simulink model "sistem_full_test"  (R2020b)
settings: Solver=ode45  StartTime=0.0  StopTime=10.0  MaxStep=0.01  RelTol=1e-3
undefined symbols (not defined in the file or in its folder): K_d, K_p, params, r_des
settings Model: Creator=Danil  LastModifiedBy=Danil

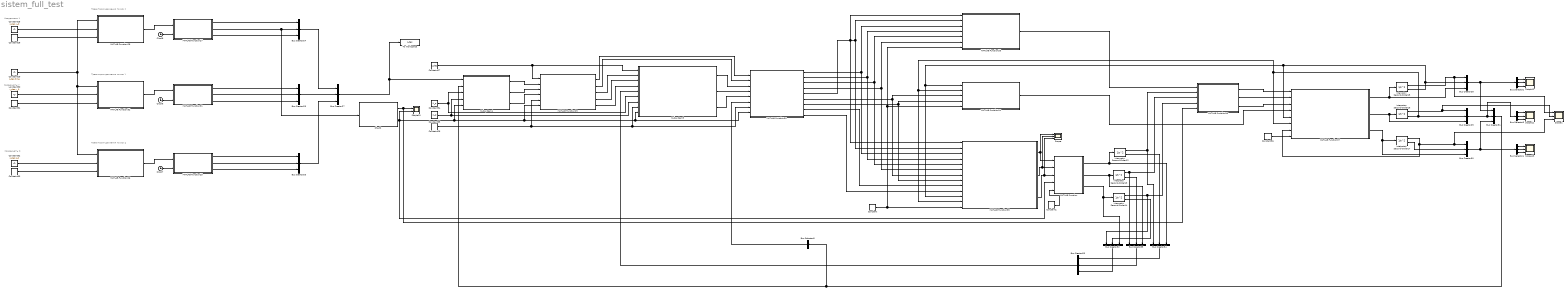
== system sistem_full_test ==
  note: Координаты X
  note: Траектория движения по оси Z
  note: Траектория движения по оси Y
  note: Траектория движения по оси X
  note: Координаты Z
  note: Координаты Y
  Bus Creator{24..35} (12 alike) : BusCreator  Inputs=3
  Bus Selector2 : BusSelector  OutputSignals=x,x_dot,x_ddot
  Bus Selector3 : BusSelector  OutputSignals=y,y_dot,y_ddot
  Bus Selector4 : BusSelector  OutputSignals=z,z_dot,z_ddot
  Bus Selector5 : BusSelector  OutputSignals=x.x_dot
  Chart2 : Stateflow chart  TreatAsAtomicUnit=on
      settings: PortSchema="{\"entries\":[{\"content\":{\"sides\":[{\"content\":{\"connectorIds\":[\"In1\"]},\"type\":\"ConnectorPlacement.EquallySpacedRectSide\",\"uuid\":\"990aaa4d-e872-427e-8bc8-a44f7de52f17\"},{\"content\":{\"connectorIds\":[\"Out2\",\"Out1\"],\"side\":\"RIGHT\"},\"type\":\"ConnectorPlacement.EquallySpacedRectSide\",\"uuid\":\"6e7ad4a8-1d47-4f26-af3c-4dfef899b5bc\"},{\"content\":{\"connectorIds\":[],\"side\":\"TOP\"},\"type\":\"ConnectorPlacement.EquallySpacedRectSide\",\"uuid\":\"20d3b10c-4783-40ca-8243-63709ccaf162\"},{\"content\":{\"connectorIds\":[],\"side\":\"HIDDEN\"},\"type\":\"ConnectorPlacement.EquallySpacedRectSide\",\"uuid\":\"c78cf433-ac9b-47b8-aa1e-24a5718d794b\"}]},\"type\":\"ConnectorPlacement.EquallySpacedConnector\",\"uuid\":\"eb598262-5703-4057-871f-faa738de211a\"}],\"packageUris\":[\"http://schema.mathworks.com/mf0/Connector/R2020b\"],\"version\":\"1.0\"}"
  Clock6 : Clock
  Clock7 : Clock
  Clock8 : Clock
  Constant{,1,26,36} (4 alike) : Constant  Value=params  OutDataTypeStr=Bus: params_bus
  Constant25 : Constant  Value=r_des.x_0
  Constant27 : Constant  Value=r_des  OutDataTypeStr=Bus: r_des_bus
  Constant28 : Constant  Value=r_des.x
  Constant29 : Constant  Value=r_des.time
  Constant30 : Constant  Value=r_des.y_0
  Constant31 : Constant  Value=r_des.y
  Constant32 : Constant  Value=r_des.z_0
  Constant33 : Constant  Value=r_des.z
  Constant34 : Constant  Value=K_p  OutDataTypeStr=Bus: K_p_bus
  Constant35 : Constant  Value=K_d  OutDataTypeStr=Bus: K_d_bus
  Integrator, Second-Order{12..17} (6 alike) : SecondOrderIntegrator
  MATLAB Function : MATLAB Function  TreatAsAtomicUnit=on
  MATLAB Function25 : MATLAB Function  TreatAsAtomicUnit=on
  MATLAB Function26 : MATLAB Function  TreatAsAtomicUnit=on
  MATLAB Function27 : MATLAB Function  TreatAsAtomicUnit=on
  MATLAB Function28 : MATLAB Function  TreatAsAtomicUnit=on
  MATLAB Function29 : MATLAB Function  TreatAsAtomicUnit=on
  MATLAB Function30 : MATLAB Function  TreatAsAtomicUnit=on
  MATLAB Function31 : MATLAB Function  TreatAsAtomicUnit=on
  MATLAB Function32 : MATLAB Function  TreatAsAtomicUnit=on
  MATLAB Function33 : MATLAB Function  TreatAsAtomicUnit=on
  MATLAB Function34 : MATLAB Function  TreatAsAtomicUnit=on
  MATLAB Function35 : MATLAB Function  TreatAsAtomicUnit=on
  MATLAB Function36 : MATLAB Function  TreatAsAtomicUnit=on
  MATLAB Function37 : MATLAB Function  TreatAsAtomicUnit=on
  Scope{,1,11..13} (5 alike) : Scope  NumInputPorts=3
  Scope10 : Scope  NumInputPorts=2
  Subsystem4 : Subsystem
  Subsystem5 : Subsystem
  To Workspace : ToWorkspace  VariableName=r_des  SaveFormat=Timeseries  SampleTime=-1
  wires:
  MATLAB Function26/1(coeff) -> MATLAB Function25/1(coeff)
  Constant31/1 -> MATLAB Function32/3(r_end)
  MATLAB Function29/5(psi_des) -> Subsystem5/4(psi_des)
  Constant27/1 -> MATLAB Function29/1(r_des), Subsystem5/1(r_des)
  MATLAB Function27/3(acc) -> Bus Creator24/3  "x_ddot"
  Bus Creator26/1 -> Bus Creator27/3  "r_z"
  Constant35/1 -> Subsystem4/4(K_d), Subsystem5/7(K_d)
  MATLAB Function27/1(pos) -> Bus Creator24/1  "x"
  MATLAB Function29/3(fi_des) -> Subsystem5/2(fi_des)
  MATLAB Function27/2(vel) -> Chart2/1(x_dot_des), Bus Creator24/2  "x_dot"
  Constant32/1 -> MATLAB Function26/2(r_0)
  Clock7/1 -> MATLAB Function25/2(clock)
  Constant34/1 -> Subsystem4/3(K_p), Subsystem5/6(K_p)
  MATLAB Function28/1(coeff) -> MATLAB Function27/1(coeff)
  Subsystem5/1(M_x) -> MATLAB Function30/3(M_x)
  Subsystem4/2(y_ddot) -> MATLAB Function29/3(y_ddot)
  Chart2/1(mode) -> Scope10/2, MATLAB Function/4(mode), MATLAB Function29/6(mode), MATLAB Function30/8(mode), Subsystem5/9(mode), Subsystem4/5(mode)
  Subsystem4/1(x_ddot) -> MATLAB Function29/2(x_ddot)
  MATLAB Function29/4(theta_des) -> Subsystem5/3(theta_des)
  Constant25/1 -> MATLAB Function28/2(r_0)
  MATLAB Function29/1(F_T) -> MATLAB Function30/1(F_T)
  Subsystem4/3(z_ddot) -> MATLAB Function29/4(z_ddot)
  MATLAB Function31/1(pos) -> Bus Creator25/1  "y"
  MATLAB Function31/3(acc) -> Bus Creator25/3  "y_ddot"
  MATLAB Function31/2(vel) -> Bus Creator25/2  "y_dot"
  Constant28/1 -> MATLAB Function28/3(r_end)
  MATLAB Function25/1(pos) -> Bus Creator26/1  "z"
  Bus Creator24/1 -> Bus Creator27/1  "r_x"
  MATLAB Function32/1(coeff) -> MATLAB Function31/1(coeff)
  MATLAB Function25/2(vel) -> Bus Creator26/2  "z_dot"
  Subsystem5/3(M_z) -> MATLAB Function30/5(M_z)
  Constant30/1 -> MATLAB Function32/2(r_0)
  Constant33/1 -> MATLAB Function26/3(r_end)
  MATLAB Function25/3(acc) -> Bus Creator26/3  "z_ddot"
  Bus Creator25/1 -> Bus Creator27/2  "r_y"
  Clock8/1 -> MATLAB Function27/2(clock)
  Bus Creator27/1 -> To Workspace/1, Subsystem4/1(r_des)
  Constant26/1 -> MATLAB Function29/5(params), Subsystem5/8(params), MATLAB Function30/7(params)
  Subsystem5/2(M_y) -> MATLAB Function30/4(M_y)
  Clock6/1 -> MATLAB Function31/2(clock)
  Constant29/1 -> MATLAB Function26/1(t), MATLAB Function32/1(t), MATLAB Function28/1(t)
  MATLAB Function29/2(Y) -> MATLAB Function30/2(Y)
  MATLAB Function/1(fi_ddot) -> "Integrator, Second-Order12"/1, Bus Creator34/3  "fi_ddot"
  MATLAB Function37/1(x_ddot) -> Bus Creator28/3, "Integrator, Second-Order15"/1
  MATLAB Function37/3(z_ddot) -> Bus Creator30/3, "Integrator, Second-Order17"/1
  MATLAB Function30/5(w) -> MATLAB Function35/2(w_R), MATLAB Function33/2(w_R), MATLAB Function33/1(w_L), MATLAB Function35/1(w_L)
  MATLAB Function/3(psi_ddot) -> Bus Creator32/3, "Integrator, Second-Order14"/1  "psi_ddot"
  MATLAB Function36/1(F_x) -> MATLAB Function37/1(F_x)
  MATLAB Function37/2(y_ddot) -> Bus Creator29/3, "Integrator, Second-Order16"/1
  MATLAB Function36/3(F_z) -> MATLAB Function37/3(F_z)
  "Integrator, Second-Order16"/2 -> MATLAB Function37/6(y_dot), MATLAB Function34/2(y_dot), MATLAB Function35/12(y_dot), Bus Creator29/2  "y_dot"
  MATLAB Function30/1(alpha_1) -> MATLAB Function35/3(alpha_1), MATLAB Function33/3(alpha_1)
  MATLAB Function30/6(alpha_L) -> MATLAB Function35/7(alpha_L), MATLAB Function34/3(alpha_L)
  MATLAB Function30/4(alpha_4) -> MATLAB Function35/6(alpha_4), MATLAB Function33/6(alpha_4)
  MATLAB Function/2(theta_ddot) -> Bus Creator35/3, "Integrator, Second-Order13"/1  "theta_ddot"
  "Integrator, Second-Order15"/2 -> Bus Creator28/2, MATLAB Function37/5(x_dot), MATLAB Function34/1(x_dot), MATLAB Function35/11(x_dot)  "x_dot"
  MATLAB Function34/1(Y) -> MATLAB Function37/4(Y)
  Constant/1 -> MATLAB Function35/13(params), MATLAB Function34/5(params), MATLAB Function33/7(params)
  Constant36/1 -> MATLAB Function37/8(params)
  "Integrator, Second-Order12"/1 -> MATLAB Function36/2(fi), Bus Creator34/1  "fi"
  MATLAB Function33/1(F) -> MATLAB Function36/1(F)
  MATLAB Function30/2(alpha_2) -> MATLAB Function35/4(alpha_2), MATLAB Function33/4(alpha_2)
  MATLAB Function30/9(alpha_F) -> MATLAB Function35/10(alpha_F)
  MATLAB Function30/8(alpha_H) -> MATLAB Function35/9(alpha_H)
  MATLAB Function36/2(F_y) -> MATLAB Function37/2(F_y)
  MATLAB Function30/7(alpha_R) -> MATLAB Function35/8(alpha_R), MATLAB Function34/4(alpha_R)
  MATLAB Function30/3(alpha_3) -> MATLAB Function35/5(alpha_3), MATLAB Function33/5(alpha_3)
  Chart2/2(sigma) -> MATLAB Function36/5(sigma), Scope10/1
  "Integrator, Second-Order14"/1 -> Bus Creator32/1, MATLAB Function36/4(psi)  "psi"
  "Integrator, Second-Order17"/1 -> Scope1/3, Bus Creator30/1, MATLAB Function37/7(z_dot)  "z"
  "Integrator, Second-Order13"/1 -> MATLAB Function36/3(theta), Bus Creator35/1  "theta"
  Bus Creator28/1 -> Bus Creator31/1, Bus Selector2/1  "x"
  Bus Creator29/1 -> Bus Selector3/1, Bus Creator31/2  "y"
  Bus Creator30/1 -> Bus Selector4/1, Bus Creator31/3  "z"
  Bus Creator32/1 -> Bus Creator33/3  "psi"
  Bus Creator34/1 -> Bus Creator33/1  "fi"
  Bus Creator35/1 -> Bus Creator33/2  "theta"
  "Integrator, Second-Order15"/1 -> Scope1/1, Bus Creator28/1  "x"
  "Integrator, Second-Order16"/1 -> Bus Creator29/1, Scope1/2  "y"
  "Integrator, Second-Order17"/2 -> Bus Creator30/2  "z_dot"
  Bus Selector3/2 -> Scope11/2  "<y_dot>"
  Bus Selector3/3 -> Scope11/3  "<y_ddot>"
  Bus Selector3/1 -> Scope11/1  "<y>"
  Bus Selector4/2 -> Scope13/2  "<z_dot>"
  Bus Selector4/3 -> Scope13/3  "<z_ddot>"
  Bus Selector4/1 -> Scope13/1  "<z>"
  Bus Selector2/2 -> Scope12/2  "<x_dot>"
  Bus Selector2/3 -> Scope12/3  "<x_ddot>"
  Bus Selector2/1 -> Scope12/1  "<x>"
  "Integrator, Second-Order12"/2 -> Bus Creator34/2  "fi_dot"
  "Integrator, Second-Order13"/2 -> Bus Creator35/2  "theta_dot"
  "Integrator, Second-Order14"/2 -> Bus Creator32/2  "psi_dot"
  Bus Creator31/1 -> Bus Selector5/1, Subsystem4/2(r)
  Bus Creator33/1 -> Subsystem5/5(r)
  Bus Selector5/1 -> MATLAB Function30/6(x_dot)  "<x_dot>"
  MATLAB Function35/1(M_x) -> MATLAB Function/1(M_x), Scope/1
  MATLAB Function35/2(M_y) -> Scope/2, MATLAB Function/2(M_y)
  MATLAB Function35/3(M_z) -> Scope/3, MATLAB Function/3(M_z)
  Constant1/1 -> MATLAB Function/5(params)

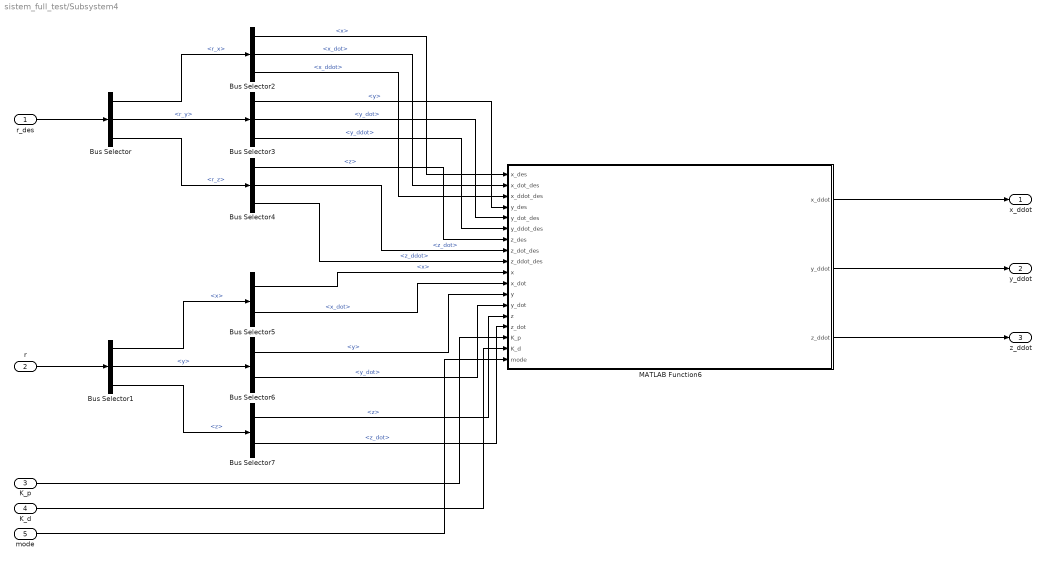
== system sistem_full_test/Subsystem4 ==
  r_des : Inport
  r : Inport  Port=2
  K_p : Inport  Port=3
  K_d : Inport  Port=4
  mode : Inport  Port=5
  Bus Selector : BusSelector  OutputSignals=r_x,r_y,r_z
  Bus Selector1 : BusSelector  OutputSignals=x,y,z
  Bus Selector2 : BusSelector  OutputSignals=x,x_dot,x_ddot
  Bus Selector3 : BusSelector  OutputSignals=y,y_dot,y_ddot
  Bus Selector4 : BusSelector  OutputSignals=z,z_dot,z_ddot
  Bus Selector5 : BusSelector  OutputSignals=x,x_dot
  Bus Selector6 : BusSelector  OutputSignals=y,y_dot
  Bus Selector7 : BusSelector  OutputSignals=z,z_dot
  MATLAB Function6 : MATLAB Function  TreatAsAtomicUnit=on
  x_ddot : Outport
  y_ddot : Outport  Port=2
  z_ddot : Outport  Port=3
  wires:
  Bus Selector3/1 -> MATLAB Function6/4(y_des)  "<y>"
  Bus Selector4/3 -> MATLAB Function6/9(z_ddot_des)  "<z_ddot>"
  Bus Selector4/1 -> MATLAB Function6/7(z_des)  "<z>"
  Bus Selector/1 -> Bus Selector2/1  "<r_x>"
  Bus Selector5/2 -> MATLAB Function6/11(x_dot)  "<x_dot>"
  Bus Selector3/2 -> MATLAB Function6/5(y_dot_des)  "<y_dot>"
  Bus Selector/3 -> Bus Selector4/1  "<r_z>"
  r/1 -> Bus Selector1/1
  r_des/1 -> Bus Selector/1
  Bus Selector2/1 -> MATLAB Function6/1(x_des)  "<x>"
  Bus Selector5/1 -> MATLAB Function6/10(x)  "<x>"
  MATLAB Function6/2(y_ddot) -> y_ddot/1
  MATLAB Function6/3(z_ddot) -> z_ddot/1
  K_d/1 -> MATLAB Function6/17(K_d)
  K_p/1 -> MATLAB Function6/16(K_p)
  Bus Selector1/3 -> Bus Selector7/1  "<z>"
  Bus Selector2/2 -> MATLAB Function6/2(x_dot_des)  "<x_dot>"
  Bus Selector7/2 -> MATLAB Function6/15(z_dot)  "<z_dot>"
  MATLAB Function6/1(x_ddot) -> x_ddot/1
  Bus Selector6/1 -> MATLAB Function6/12(y)  "<y>"
  Bus Selector7/1 -> MATLAB Function6/14(z)  "<z>"
  Bus Selector4/2 -> MATLAB Function6/8(z_dot_des)  "<z_dot>"
  Bus Selector2/3 -> MATLAB Function6/3(x_ddot_des)  "<x_ddot>"
  Bus Selector1/1 -> Bus Selector5/1  "<x>"
  Bus Selector1/2 -> Bus Selector6/1  "<y>"
  Bus Selector6/2 -> MATLAB Function6/13(y_dot)  "<y_dot>"
  Bus Selector3/3 -> MATLAB Function6/6(y_ddot_des)  "<y_ddot>"
  Bus Selector/2 -> Bus Selector3/1  "<r_y>"
  mode/1 -> MATLAB Function6/18(mode)

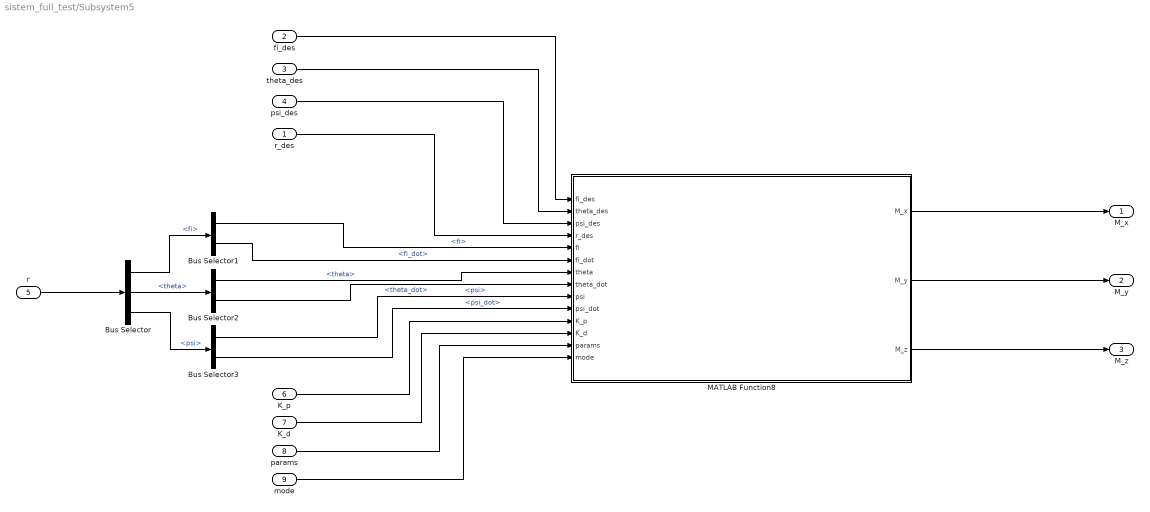
== system sistem_full_test/Subsystem5 ==
  r_des : Inport
  fi_des : Inport  Port=2
  theta_des : Inport  Port=3
  psi_des : Inport  Port=4
  r : Inport  Port=5
  K_p : Inport  Port=6
  K_d : Inport  Port=7
  params : Inport  Port=8
  mode : Inport  Port=9
  Bus Selector : BusSelector  OutputSignals=fi,theta,psi
  Bus Selector1 : BusSelector  OutputSignals=fi,fi_dot
  Bus Selector2 : BusSelector  OutputSignals=theta,theta_dot
  Bus Selector3 : BusSelector  OutputSignals=psi,psi_dot
  MATLAB Function8 : MATLAB Function  TreatAsAtomicUnit=on
  M_x : Outport
  M_y : Outport  Port=2
  M_z : Outport  Port=3
  wires:
  Bus Selector3/1 -> MATLAB Function8/9(psi)  "<psi>"
  Bus Selector1/2 -> MATLAB Function8/6(fi_dot)  "<fi_dot>"
  Bus Selector/1 -> Bus Selector1/1  "<fi>"
  Bus Selector1/1 -> MATLAB Function8/5(fi)  "<fi>"
  r/1 -> Bus Selector/1
  MATLAB Function8/3(M_z) -> M_z/1
  MATLAB Function8/1(M_x) -> M_x/1
  MATLAB Function8/2(M_y) -> M_y/1
  Bus Selector2/2 -> MATLAB Function8/8(theta_dot)  "<theta_dot>"
  K_p/1 -> MATLAB Function8/11(K_p)
  Bus Selector2/1 -> MATLAB Function8/7(theta)  "<theta>"
  Bus Selector/2 -> Bus Selector2/1  "<theta>"
  r_des/1 -> MATLAB Function8/4(r_des)
  params/1 -> MATLAB Function8/13(params)
  psi_des/1 -> MATLAB Function8/3(psi_des)
  fi_des/1 -> MATLAB Function8/1(fi_des)
  K_d/1 -> MATLAB Function8/12(K_d)
  theta_des/1 -> MATLAB Function8/2(theta_des)
  Bus Selector3/2 -> MATLAB Function8/10(psi_dot)  "<psi_dot>"
  Bus Selector/3 -> Bus Selector3/1  "<psi>"
  mode/1 -> MATLAB Function8/14(mode)

== matlab function sistem_full_test/MATLAB Function30 ==
  data: alpha_1 output; alpha_2 output; alpha_3 output; alpha_4 output; F_T input; Y input; w output; M_x input; M_y input; M_z input; x_dot input; params input; alpha_L output; alpha_R output; alpha_H output; alpha_F output; mode input
function [alpha_1, alpha_2, alpha_3, alpha_4, w, alpha_L, alpha_R, alpha_H, alpha_F] = fcn(F_T, Y, M_x, M_y, M_z, x_dot, params, mode)

if mode == 0
    
    alpha_1 = (1 / (4 * params.k_Y)) * (F_T + M_x + M_y + M_z) - 7;
    alpha_2 = (1 / (4 * params.k_Y)) * (F_T + M_x - M_y - M_z);
    alpha_3 = (1 / (4 * params.k_Y)) * (F_T - M_x + M_y - M_z) - 7;
    alpha_4 = (1 / (4 * params.k_Y)) * (F_T - M_x - M_y + M_z);
    
    w = params.w_0;
    alpha_L = -7;
    alpha_R = -7;
    alpha_H = 0;
    alpha_F = 0;
    
elseif mode == 1
    
    alpha_1 = 7.5;
    alpha_2 = 7.5;
    alpha_3 = 7.5;
    alpha_4 = 7.5;

    w = (50000 * F_T + 245100) / 77;

    alpha_L = (500 * M_x + 500 * Y + 102201 * params.S_k * params.rho - 14630 * params.S_k * params.rho * x_dot) / (30 * params.S_k * params.rho * (70 * x_dot - 489));
    alpha_R = - (500 * M_x - 500 * Y - 102201 * params.S_k * params.rho + 14630 * params.S_k * params.rho * x_dot) / (30 * params.S_k * params.rho * (70 * x_dot - 489));
    alpha_H = (125 * M_y) / (3 * params.S_h * params.rho * (70 * x_dot - 489));
    alpha_F = (125 * M_z) / (3 * params.S_f * params.rho * (70 * x_dot - 489));
    
else
    
    alpha_1 = (1 / (4 * params.k_Y)) * (F_T + M_x + M_y + M_z) - 7;
    alpha_2 = (1 / (4 * params.k_Y)) * (F_T + M_x - M_y - M_z);
    alpha_3 = (1 / (4 * params.k_Y)) * (F_T - M_x + M_y - M_z) - 7;
    alpha_4 = (1 / (4 * params.k_Y)) * (F_T - M_x - M_y + M_z);
    
    w = params.w_0;
    alpha_L = -7;
    alpha_R = -7;
    alpha_H = 0;
    alpha_F = 0;
    
end

== matlab function sistem_full_test/MATLAB Function31 ==
  data: coeff input; pos output; clock input; vel output; acc output
function [pos, vel, acc] = trajectories_calculation(coeff, clock)

T_p = [clock^5      clock^4     clock^3     clock^2     clock   1]';
T_v = [5*clock^4    4*clock^3   3*clock^2   2*clock     1       0]';
T_a = [20*clock^3   12*clock^2  6*clock     2           0       0]';

pos = sum(coeff.*T_p);
vel = sum(coeff.*T_v);
acc = sum(coeff.*T_a);

== matlab function sistem_full_test/MATLAB Function32 ==
  data: t input; coeff output; r_0 input; r_end input
function coeff  = calculation_coefficients(t, r_0, r_end)

x_0 = r_0;
x_dot_0 = 0;
x_ddot_0 = 0;

x_des = r_end;
x_dot_des = 0;
x_ddot_des = 0;

waypoints = [x_0    x_dot_0     x_ddot_0;
             x_des  x_dot_des   x_ddot_des]';
t = [0 t];

time_size = size(t);
n = 0;
%T = linspace(0, time_size(2) - 1, point(2));


border_conditions_sigm = reshape(waypoints(:, n + 1 : n + 2),1,[]);
%disp(border_conditions_sigm)

coeff = zeros(6, 1);

parameters = [1 * (t(n + 1) ^ 5), 1 * (t(n + 1) ^ 4), 1 * (t(n + 1) ^ 3), 1 * (t(n + 1) ^ 2), 1 * (t(n + 1) ^ 1), 1 * (t(n + 1) ^ 0);
              5 * (t(n + 1) ^ 4), 4 * (t(n + 1) ^ 3), 3 * (t(n + 1) ^ 2), 2 * (t(n + 1) ^ 1), 1 * (t(n + 1) ^ 0), 0 * (t(n + 1) ^ 0);
              20 * (t(n + 1) ^ 3), 12 * (t(n + 1) ^ 2), 6 * (t(n + 1) ^ 1), 2 * (t(n + 1) ^ 0), 0 * (t(n + 1) ^ 0), 0 * (t(n + 1) ^ 0);
              1 * (t(n + 2) ^ 5), 1 * (t(n + 2) ^ 4), 1 * (t(n + 2) ^ 3), 1 * (t(n + 2) ^ 2), 1 * (t(n + 2) ^ 1), 1 * (t(n + 2) ^ 0);
              5 * (t(n + 2) ^ 4), 4 * (t(n + 2) ^ 3), 3 * (t(n + 2) ^ 2), 2 * (t(n + 2) ^ 1), 1 * (t(n + 2) ^ 0), 0 * (t(n + 2) ^ 0);
              20 * (t(n + 2) ^ 3), 12 * (t(n + 2) ^ 2), 6 * (t(n + 2) ^ 1), 2 * (t(n + 2) ^ 0), 0 * (t(n + 2) ^ 0), 0 * (t(n + 2) ^ 0)];

coeff = inv(parameters) * border_conditions_sigm';

== matlab function sistem_full_test/Subsystem4/MATLAB Function6 ==
  data: x_des input; x_ddot output; x_dot_des input; x_ddot_des input; y_des input; y_dot_des input; y_ddot_des input; z_des input; z_dot_des input; z_ddot_des input; x input; x_dot input; y input; y_dot input; z input; z_dot input; K_p input; K_d input; y_ddot output; z_ddot output; mode input
function [x_ddot,y_ddot,z_ddot] = fcn(x_des, x_dot_des, x_ddot_des, y_des, y_dot_des, y_ddot_des, z_des, z_dot_des, z_ddot_des, ...
                                      x, x_dot, y, y_dot, z, z_dot, K_p, K_d, mode)

if mode == 0
    
    x_ddot = x_ddot_des + abs(K_d.ver.x) * (x_dot_des - x_dot) + abs(K_p.ver.x) * (x_des - x);
    y_ddot = y_ddot_des + abs(K_d.ver.y) * (y_dot_des - y_dot) + abs(K_p.ver.y) * (y_des - y);
    z_ddot = z_ddot_des + abs(K_d.ver.z) * (z_dot_des - z_dot) + abs(K_p.ver.z) * (z_des - z);

elseif mode == 1
    
    x_ddot = x_ddot_des + abs(K_d.hor.x) * (x_dot_des - x_dot) + abs(K_p.hor.x) * (x_des - x);
    y_ddot = y_ddot_des + abs(K_d.hor.y) * (y_dot_des - y_dot) + abs(K_p.hor.y) * (y_des - y);
    z_ddot = z_ddot_des + abs(K_d.hor.z) * (z_dot_des - z_dot) + abs(K_p.hor.z) * (z_des - z);
    
else
    
    x_ddot = x_ddot_des + abs(K_d.ver.x) * (x_dot_des - x_dot) + abs(K_p.ver.x) * (x_des - x);
    y_ddot = y_ddot_des + abs(K_d.ver.y) * (y_dot_des - y_dot) + abs(K_p.ver.y) * (y_des - y);
    z_ddot = z_ddot_des + abs(K_d.ver.z) * (z_dot_des - z_dot) + abs(K_p.ver.z) * (z_des - z);
    
end

== matlab function sistem_full_test/Subsystem5/MATLAB Function8 ==
  data: fi_des input; theta_des input; psi_des input; r_des input; fi input; fi_dot input; theta input; theta_dot input; psi input; psi_dot input; M_x output; K_p input; K_d input; params input; M_y output; M_z output; mode input
function [M_x, M_y, M_z] = fcn(fi_des, theta_des, psi_des, r_des, fi, fi_dot, theta, theta_dot, psi, psi_dot, K_p, K_d, params, mode)

if mode == 0

    M_x = (params.ver.J_xx / params.ver.L_x) * (r_des.fi_ddot + abs(K_d.ver.fi) * (r_des.fi_dot - fi_dot) + abs(K_p.ver.fi) * (fi_des - fi));
    M_y = (params.ver.J_yy / params.ver.L_y) * (r_des.theta_ddot + abs(K_d.ver.theta) * (r_des.theta_dot - theta_dot) + abs(K_p.ver.theta) * (theta_des - theta));
    M_z = (params.ver.J_zz / params.ver.L_z) * (r_des.psi_ddot + abs(K_d.ver.psi) * (r_des.psi_dot - psi_dot) + abs(K_p.ver.psi) * (psi_des - psi));
    
elseif mode == 1
    
    M_x = (params.hor.J_xx / params.hor.L_x) * (r_des.fi_ddot + abs(K_d.hor.fi) * (r_des.fi_dot - fi_dot) + abs(K_p.hor.fi) * (fi_des - fi));
    M_y = (params.hor.J_yy / params.hor.L_y) * (r_des.theta_ddot + abs(K_d.hor.theta) * (r_des.theta_dot - theta_dot) + abs(K_p.hor.theta) * (theta_des - theta));
    M_z = (params.hor.J_zz / params.hor.L_z) * (r_des.psi_ddot + abs(K_d.hor.psi) * (r_des.psi_dot - psi_dot) + abs(K_p.hor.psi) * (psi_des - psi));
    
else 
    
    M_x = (params.ver.J_xx / params.ver.L_x) * (r_des.fi_ddot + abs(K_d.ver.fi) * (r_des.fi_dot - fi_dot) + abs(K_p.ver.fi) * (fi_des - fi));
    M_y = (params.ver.J_yy / params.ver.L_y) * (r_des.theta_ddot + abs(K_d.ver.theta) * (r_des.theta_dot - theta_dot) + abs(K_p.ver.theta) * (theta_des - theta));
    M_z = (params.ver.J_zz / params.ver.L_z) * (r_des.psi_ddot + abs(K_d.ver.psi) * (r_des.psi_dot - psi_dot) + abs(K_p.ver.psi) * (psi_des - psi));
    
end

== matlab function sistem_full_test/MATLAB Function33 ==
  data: w_L input; F output; w_R input; alpha_1 input; alpha_2 input; alpha_3 input; alpha_4 input; params input
function F  = fcn(w_L, w_R, alpha_1, alpha_2, alpha_3, alpha_4, params)

alpha_L = alpha_1 + alpha_2;
alpha_R = alpha_3 + alpha_4;

C_Y_L = params.a_l * alpha_L^2 + params.b_l * alpha_L + params.c_l;
C_Y_R = params.a_l * alpha_R^2 + params.b_l * alpha_R + params.c_l;

F = (3/2) * params.rho * params.S_l * (C_Y_L * w_L^2 + C_Y_R * w_R^2);

== matlab function sistem_full_test/MATLAB Function34 ==
  data: x_dot input; y_dot input; alpha_L input; alpha_R input; params input; Y output
function Y = fcn(x_dot, y_dot, alpha_L, alpha_R, params)

C_y_L = params.a_k * alpha_L^2 + params.b_k * alpha_L + params.c_k;
C_y_R = params.a_k * alpha_R^2 + params.b_k * alpha_R + params.c_k;

Y = (1 / 2) * params.rho * (x_dot^2 + y_dot^2) * params.S_k * (C_y_L + C_y_R);

== matlab function sistem_full_test/MATLAB Function35 ==
  data: w_L input; w_R input; alpha_1 input; alpha_2 input; alpha_3 input; alpha_4 input; alpha_L input; alpha_R input; alpha_H input; alpha_F input; x_dot input; y_dot input; M_x output; M_y output; M_z output; params input
function [M_x, M_y, M_z] = fcn(w_L, w_R, alpha_1, alpha_2, alpha_3, alpha_4, ...
                               alpha_L, alpha_R, alpha_H, alpha_F, x_dot, y_dot, params)

C_y_L_l_x = params.a_l * (alpha_1 + alpha_2)^2 + params.b_l * (alpha_1 + alpha_2) + params.c_l;
C_y_R_l_x = params.a_l * (alpha_3 + alpha_4)^2 + params.b_l * (alpha_3 + alpha_4) + params.c_l;

C_y_L_l_yz = params.a_l * (alpha_1 - alpha_2)^2 + params.b_l * (alpha_1 - alpha_2) + params.c_l;
C_y_R_l_yz = params.a_l * (alpha_3 - alpha_4)^2 + params.b_l * (alpha_3 - alpha_4) + params.c_l;

C_y_L_k = params.a_k * alpha_L^2 + params.b_k * alpha_L + params.c_k;
C_y_R_k = params.a_k * alpha_R^2 + params.b_k * alpha_R + params.c_k;

C_y_H = params.a_h * alpha_H^3 + params.b_h * alpha_H^2 + params.c_h * alpha_H + params.d_h;
C_y_F = params.a_f * alpha_F^3 + params.b_f * alpha_F^2 + params.c_f * alpha_F + params.d_f;

M_x = ((3 / 2) * params.rho * params.S_l * (C_y_L_l_x * w_L^2 - C_y_R_l_x * w_R^2)) + ...
      ((1 / 2) * params.rho * params.S_k * (x_dot^2 + y_dot^2) * (C_y_L_k - C_y_R_k));
  
M_y = ((3 / 2) * params.rho * params.S_l * (C_y_L_l_yz * w_L^2 + C_y_R_l_yz * w_R^2)) + ...
      ((1 / 2) * C_y_H * params.rho * params.S_h * (x_dot^2 + y_dot^2));
  
M_z = ((3 / 2) * params.rho * params.S_l * (C_y_L_l_yz * w_L^2 - C_y_R_l_yz * w_R^2)) + ...
      ((1 / 2) * C_y_F * params.rho * params.S_f * (x_dot^2 + y_dot^2));

== matlab function sistem_full_test/MATLAB Function36 ==
  data: F input; F_x output; fi input; theta input; psi input; F_y output; F_z output; sigma input
function [F_x, F_y, F_z] = fcn(F, fi, theta, psi, sigma)

sigma = sigma * pi / 180;

F_x = F * sin(sigma) * (cos(psi) * sin(theta) + cos(theta) * sin(fi) * sin(psi)) + F * cos(sigma) * (cos(psi) * cos(theta));
F_y = F * sin(sigma) * (sin(psi) * sin(theta) - cos(psi) * cos(theta) * sin(fi)) + F * cos(sigma) * (cos(fi) * sin(psi) + cos(psi) * sin(fi) * sin(theta));
F_z = F * sin(sigma) * (cos(fi) * cos(theta)) + F * cos(sigma) * (sin(fi) * sin(psi) - cos(fi) * cos(psi) * sin(theta));

== matlab function sistem_full_test/MATLAB Function37 ==
  data: F_x input; x_ddot output; F_y input; F_z input; Y input; x_dot input; y_dot input; z_dot input; params input; y_ddot output; z_ddot output
function [x_ddot, y_ddot, z_ddot] = fcn(F_x, F_y, F_z, Y, x_dot, y_dot, z_dot, params)

x_ddot = (1 / params.m) * (F_x - params.k_x * x_dot);
y_ddot = (1 / params.m) * (F_y - params.k_y * y_dot);
z_ddot = (1 / params.m) * (F_z + Y - params.k_z * z_dot - params.m * params.g);

== matlab function sistem_full_test/MATLAB Function ==
  data: M_x input; fi_ddot output; M_y input; M_z input; mode input; params input; theta_ddot output; psi_ddot output
function [fi_ddot, theta_ddot, psi_ddot] = fcn(M_x, M_y, M_z, mode, params)

if mode == 0
    
    fi_ddot = (params.ver.L_x / params.ver.J_xx) * M_x;
    theta_ddot = (params.ver.L_y / params.ver.J_yy) * M_y;
    psi_ddot = (params.ver.L_z / params.ver.J_zz) * M_z;
    
elseif mode == 1
    
    fi_ddot = (params.hor.L_x / params.hor.J_xx) * M_x;
    theta_ddot = (params.hor.L_y / params.hor.J_yy) * M_y;
    psi_ddot = (params.hor.L_z / params.hor.J_zz) * M_z;
    
else
    
    fi_ddot = (params.ver.L_x / params.ver.J_xx) * M_x;
    theta_ddot = (params.ver.L_y / params.ver.J_yy) * M_y;
    psi_ddot = (params.ver.L_z / params.ver.J_zz) * M_z;
    
end

== stateflow chart sistem_full_test/Chart2 ==
  state Vertical_flight
    mode = 0
    sigma = 90
  state Horizontal_flight
    mode = 1
    sigma = 0
  (default) -> Vertical_flight
  Horizontal_flight -> Vertical_flight : [x_dot_des < 14.1]
  Vertical_flight -> Horizontal_flight : [x_dot_des > 14.1]
  data: mode output; x_dot_des input; sigma output

== matlab function sistem_full_test/MATLAB Function25 ==
  data: coeff input; pos output; clock input; vel output; acc output
function [pos, vel, acc] = trajectories_calculation(coeff, clock)

T_p = [clock^5      clock^4     clock^3     clock^2     clock   1]';
T_v = [5*clock^4    4*clock^3   3*clock^2   2*clock     1       0]';
T_a = [20*clock^3   12*clock^2  6*clock     2           0       0]';

pos = sum(coeff.*T_p);
vel = sum(coeff.*T_v);
acc = sum(coeff.*T_a);

== matlab function sistem_full_test/MATLAB Function26 ==
  data: t input; coeff output; r_0 input; r_end input
function coeff  = calculation_coefficients(t, r_0, r_end)

x_0 = r_0;
x_dot_0 = 0;
x_ddot_0 = 0;

x_des = r_end;
x_dot_des = 0;
x_ddot_des = 0;

waypoints = [x_0    x_dot_0     x_ddot_0;
             x_des  x_dot_des   x_ddot_des]';
t = [0 t];

time_size = size(t);
n = 0;
%T = linspace(0, time_size(2) - 1, point(2));


border_conditions_sigm = reshape(waypoints(:, n + 1 : n + 2),1,[]);
%disp(border_conditions_sigm)

coeff = zeros(6, 1);

parameters = [1 * (t(n + 1) ^ 5), 1 * (t(n + 1) ^ 4), 1 * (t(n + 1) ^ 3), 1 * (t(n + 1) ^ 2), 1 * (t(n + 1) ^ 1), 1 * (t(n + 1) ^ 0);
              5 * (t(n + 1) ^ 4), 4 * (t(n + 1) ^ 3), 3 * (t(n + 1) ^ 2), 2 * (t(n + 1) ^ 1), 1 * (t(n + 1) ^ 0), 0 * (t(n + 1) ^ 0);
              20 * (t(n + 1) ^ 3), 12 * (t(n + 1) ^ 2), 6 * (t(n + 1) ^ 1), 2 * (t(n + 1) ^ 0), 0 * (t(n + 1) ^ 0), 0 * (t(n + 1) ^ 0);
              1 * (t(n + 2) ^ 5), 1 * (t(n + 2) ^ 4), 1 * (t(n + 2) ^ 3), 1 * (t(n + 2) ^ 2), 1 * (t(n + 2) ^ 1), 1 * (t(n + 2) ^ 0);
              5 * (t(n + 2) ^ 4), 4 * (t(n + 2) ^ 3), 3 * (t(n + 2) ^ 2), 2 * (t(n + 2) ^ 1), 1 * (t(n + 2) ^ 0), 0 * (t(n + 2) ^ 0);
              20 * (t(n + 2) ^ 3), 12 * (t(n + 2) ^ 2), 6 * (t(n + 2) ^ 1), 2 * (t(n + 2) ^ 0), 0 * (t(n + 2) ^ 0), 0 * (t(n + 2) ^ 0)];

coeff = inv(parameters) * border_conditions_sigm';

== matlab function sistem_full_test/MATLAB Function27 ==
  data: coeff input; pos output; clock input; vel output; acc output
function [pos, vel, acc] = trajectories_calculation(coeff, clock)

T_p = [clock^5      clock^4     clock^3     clock^2     clock   1]';
T_v = [5*clock^4    4*clock^3   3*clock^2   2*clock     1       0]';
T_a = [20*clock^3   12*clock^2  6*clock     2           0       0]';

pos = sum(coeff.*T_p);
vel = sum(coeff.*T_v);
acc = sum(coeff.*T_a);

== matlab function sistem_full_test/MATLAB Function28 ==
  data: t input; coeff output; r_0 input; r_end input
function coeff  = calculation_coefficients(t, r_0, r_end)

x_0 = r_0;
x_dot_0 = 0;
x_ddot_0 = 0;

x_des = r_end;
x_dot_des = 0;
x_ddot_des = 0;

waypoints = [x_0    x_dot_0     x_ddot_0;
             x_des  x_dot_des   x_ddot_des]';
t = [0 t];

time_size = size(t);
n = 0;
%T = linspace(0, time_size(2) - 1, point(2));


border_conditions_sigm = reshape(waypoints(:, n + 1 : n + 2),1,[]);
%disp(border_conditions_sigm)

coeff = zeros(6, 1);

parameters = [1 * (t(n + 1) ^ 5), 1 * (t(n + 1) ^ 4), 1 * (t(n + 1) ^ 3), 1 * (t(n + 1) ^ 2), 1 * (t(n + 1) ^ 1), 1 * (t(n + 1) ^ 0);
              5 * (t(n + 1) ^ 4), 4 * (t(n + 1) ^ 3), 3 * (t(n + 1) ^ 2), 2 * (t(n + 1) ^ 1), 1 * (t(n + 1) ^ 0), 0 * (t(n + 1) ^ 0);
              20 * (t(n + 1) ^ 3), 12 * (t(n + 1) ^ 2), 6 * (t(n + 1) ^ 1), 2 * (t(n + 1) ^ 0), 0 * (t(n + 1) ^ 0), 0 * (t(n + 1) ^ 0);
              1 * (t(n + 2) ^ 5), 1 * (t(n + 2) ^ 4), 1 * (t(n + 2) ^ 3), 1 * (t(n + 2) ^ 2), 1 * (t(n + 2) ^ 1), 1 * (t(n + 2) ^ 0);
              5 * (t(n + 2) ^ 4), 4 * (t(n + 2) ^ 3), 3 * (t(n + 2) ^ 2), 2 * (t(n + 2) ^ 1), 1 * (t(n + 2) ^ 0), 0 * (t(n + 2) ^ 0);
              20 * (t(n + 2) ^ 3), 12 * (t(n + 2) ^ 2), 6 * (t(n + 2) ^ 1), 2 * (t(n + 2) ^ 0), 0 * (t(n + 2) ^ 0), 0 * (t(n + 2) ^ 0)];

coeff = inv(parameters) * border_conditions_sigm';

== matlab function sistem_full_test/MATLAB Function29 ==
  data: r_des input; F_T output; Y output; fi_des output; x_ddot input; y_ddot input; z_ddot input; params input; mode input; theta_des output; psi_des output
function [F_T, Y, fi_des, theta_des, psi_des] = fcn(r_des, x_ddot, y_ddot, z_ddot, params, mode)

if mode == 0
    
    F_T = params.m * (z_ddot + params.g);
    Y = 0;

    fi_des = (1 / params.g) * (x_ddot * sin(r_des.psi) - y_ddot * cos(r_des.psi));
    theta_des = (1 / params.g) * (x_ddot * cos(r_des.psi) + y_ddot * sin(r_des.psi));
    psi_des = r_des.psi;
    
elseif mode == 1
    
    %F_T = params.m * x_ddot + params.k_x * x_dot;

    F_T = params.m * x_ddot + r_des.x_dot;
    Y = params.m * params.g;

    fi_des = r_des.fi;
    theta_des = (params.m / (params.k_x * r_des.x_dot)) * (y_ddot * sin(r_des.fi) - z_ddot * cos(r_des.fi));
    psi_des = (params.m / (params.k_x * r_des.x_dot)) * (y_ddot * cos(r_des.fi) + z_ddot * sin(r_des.fi));

    %theta_des = (params.m / F_T) * (y_ddot * sin(r_des.fi) - z_ddot * cos(r_des.fi));
    %psi_des = (params.m / F_T) * (y_ddot * cos(r_des.fi) + z_ddot * sin(r_des.fi));
    
else 
    
    F_T = params.m * (z_ddot + params.g);
    Y = 0;

    fi_des = (1 / params.g) * (x_ddot * sin(r_des.psi) - y_ddot * cos(r_des.psi));
    theta_des = (1 / params.g) * (x_ddot * cos(r_des.psi) + y_ddot * sin(r_des.psi));
    psi_des = r_des.psi;
    
end
